simulink model "TCS"  (R2020a)
settings: Solver=VariableStepAuto  StartTime=0.0  StopTime=10.0  RelTol=1e-3
libraries: simulink x1
settings Model: Creator=Administrator  LastModifiedBy=Administrator

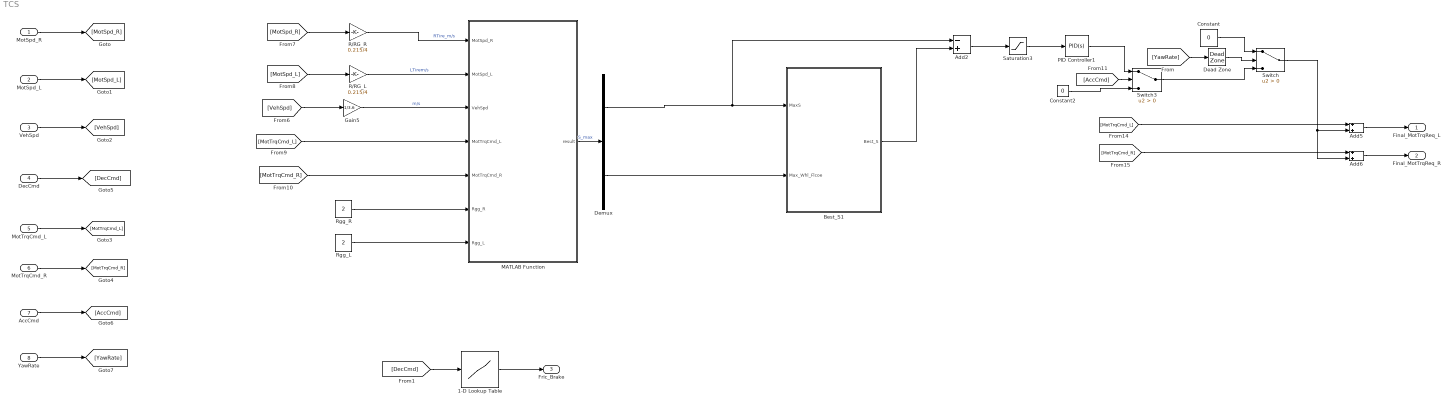
== system TCS ==
  MotSpd_R : Inport
  MotSpd_L : Inport  Port=2
  VehSpd : Inport  Port=3
  DecCmd : Inport  Port=4
  MotTrqCmd_L : Inport  Port=5
  MotTrqCmd_R : Inport  Port=6
  AccCmd : Inport  Port=7
  YawRate : Inport  Port=8
  1-D Lookup Table : Lookup_n-D  NumberOfTableDimensions=1  BreakpointsForDimension1=[0 , 0.2,0.4,0.6,0.8,1.0]  Table=[0 , 0.2,0.4,0.6,0.8,1.0]*60  InternalRulePriority=Speed  RndMeth=Simplest  InputSameDT=on
  Add2 : Sum  Inputs=-+
  Add5 : Sum
  Add6 : Sum
  Best_S1 : Subsystem
  Constant : Constant  Value=0
  Constant2 : Constant  Value=0
  Dead Zone : DeadZone  LowerValue=-0.25  UpperValue=0.25  SaturateOnIntegerOverflow=on
  Demux : Demux  Outputs=2
  Gain5 : Gain  Gain=1/3.6
  MATLAB Function : MATLAB Function  TreatAsAtomicUnit=on
  PID Controller1 : simulink/Continuous/PID Controller  Controller=PID  Form=Parallel  TimeDomain=Continuous-time  UseExternalTs=off  SampleTime=-1  IntegratorMethod=Forward Euler  FilterMethod=Forward Euler  ControllerParametersSource=internal  P=31  I=1  D=0  UseFilter=on  N=100  TunerSelectOption=Transfer Function Based (PID Tuner App)  InitialConditionSource=internal  InitialConditionForIntegrator=0  InitialConditionForFilter=0  DifferentiatorICPrevScaledInput=0  ExternalReset=none  TrackingMode=off  Kt=1  LimitOutput=off  UpperSaturationLimit=inf  LowerSaturationLimit=-inf  LinearizeAsGain=on  AntiWindupMode=none  Kb=1  POutMin=[]  POutMax=[]  IOutMin=[]  IOutMax=[]  DOutMin=[]  DOutMax=[]  NOutMin=[]  NOutMax=[]  SumOutMin=[]  SumOutMax=[]  SaturationOutMin=[]  SaturationOutMax=[]  PParamMin=[]  PParamMax=[]  IParamMin=[]  IParamMax=[]  DParamMin=[]  DParamMax=[]  NParamMin=[]  NParamMax=[]  KbParamMin=[]  KbParamMax=[]  KtParamMin=[]  KtParamMax=[]  KbOutMin=[]  KbOutMax=[]  KtOutMin=[]  KtOutMax=[]  IntegratorOutMin=[]  IntegratorOutMax=[]  FilterOutMin=[]  FilterOutMax=[]  SumI1OutMin=[]  SumI1OutMax=[]  SumI2OutMin=[]  SumI2OutMax=[]  SumI3OutMin=[]  SumI3OutMax=[]  SumI4OutMin=[]  SumI4OutMax=[]  SumDOutMin=[]  SumDOutMax=[]  DifferentiatorOutMin=[]  DifferentiatorOutMax=[]  FilterDiffOutCoefMin=[]  FilterDiffOutCoefMax=[]  ReciprocalOutMin=[]  ReciprocalOutMax=[]  SumDenOutMin=[]  SumDenOutMax=[]  SumNumOutMin=[]  SumNumOutMax=[]  DivideOutMin=[]  DivideOutMax=[]  UdiffTsProdOutMin=[]  UdiffTsProdOutMax=[]  NTsProdOutMin=[]  NTsProdOutMax=[]  UintegralTsProdOutMin=[]  UintegralTsProdOutMax=[]  UngainTsProdOutMin=[]  UngainTsProdOutMax=[]  IntegratorContinuousStateAttributes=''  IntegratorStateMustResolveToSignalObject=off  IntegratorRTWStateStorageClass=Auto  FilterContinuousStateAttributes=''  FilterStateMustResolveToSignalObject=off  FilterRTWStateStorageClass=Auto  ParallelPVariant=InternalParameters  IdealPVariant=Disabled  IVariant=InternalParameters  DVariant=InternalParameters  IntegratorVariant=Continuous  SatVariant=Disabled  AWVariant=Passthrough  PCopyVariant=Disabled  TRVariant=Disabled  FdbkBlocksVariant=Forward  IdealPFdbkVariant=Disabled  SatFdbkVariant=Disabled  DerivativeFilterVariant=ContFilter  NVariant=InternalParameters  NCopyVariant=Disabled  FilterICVariant=InternalICsFilter  IntegratorICVariant=InternalICs  ExternalResetVariant=Disabled  TRSumVariant=Passthrough  SumFdbkVariant=Disabled  SumVariant=Sum_PID  TsampFilterVariant=InternalTs  TsampNgainVariant=Passthrough  TsampIntegralVariant=Passthrough
  R/RG_L : Gain  Gain=0.215/4
  R/RG_R : Gain  Gain=0.215/4
  Rgg_L : Constant  Value=2
  Rgg_R : Constant  Value=2
  Saturation3 : Saturate  UpperLimit=2  LowerLimit=-2
  Switch : Switch  Criteria=u2 > Threshold
  Switch3 : Switch  Criteria=u2 > Threshold
  Final_MotTrqReq_L : Outport
  Final_MotTrqReq_R : Outport  Port=2
  Fric_Brake : Outport  Port=3
  wires:
  MotSpd_R/1 -> [MotSpd_R]
  MotSpd_L/1 -> [MotSpd_L]
  VehSpd/1 -> [VehSpd]
  MotTrqCmd_L/1 -> [MotTrqCmd_L]
  MotTrqCmd_R/1 -> [MotTrqCmd_R]
  DecCmd/1 -> [DecCmd]
  [VehSpd] -> Gain5/1
  [MotSpd_R] -> R/RG_R/1
  [MotSpd_L] -> R/RG_L/1
  R/RG_R/1 -> MATLAB Function/1(MotSpd_R)  "RTire_m/s"
  Gain5/1 -> MATLAB Function/3(VehSpd)  "m/s"
  R/RG_L/1 -> MATLAB Function/2(MotSpd_L)  "LTirem/s"
  Rgg_R/1 -> MATLAB Function/6(Rgg_R)
  Rgg_L/1 -> MATLAB Function/7(Rgg_L)
  [MotTrqCmd_L] -> MATLAB Function/4(MotTrqCmd_L)
  [MotTrqCmd_R] -> MATLAB Function/5(MotTrqCmd_R)
  Best_S1/1(Best_S) -> Add2/2
  Add2/1 -> Saturation3/1
  Saturation3/1 -> PID Controller1/1
  AccCmd/1 -> [AccCmd]
  [AccCmd] -> Switch3/2
  PID Controller1/1 -> Switch3/1
  Constant2/1 -> Switch3/3
  [MotTrqCmd_L] -> Add5/1
  [MotTrqCmd_R] -> Add6/1
  Add5/1 -> Final_MotTrqReq_L/1
  Add6/1 -> Final_MotTrqReq_R/1
  YawRate/1 -> [YawRate]
  Switch3/1 -> Switch/3
  Constant/1 -> Switch/1
  Switch/1 -> Add5/2, Add6/2
  [YawRate] -> Dead Zone/1
  Dead Zone/1 -> Switch/2
  1-D Lookup Table/1 -> Fric_Brake/1
  [DecCmd] -> 1-D Lookup Table/1
  MATLAB Function/1(result) -> Demux/1  "S_max"
  Demux/1 -> Add2/1, Best_S1/1(MaxS)
  Demux/2 -> Best_S1/2(Max_Whl_Flcoe)

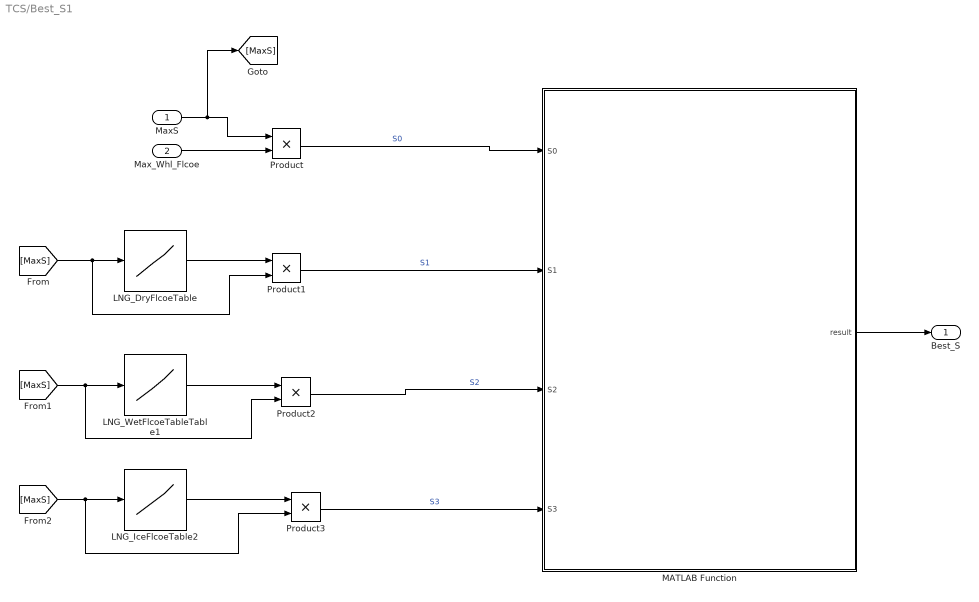
== system TCS/Best_S1 ==
  MaxS : Inport
  Max_Whl_Flcoe : Inport  Port=2
  LNG_DryFlcoeTable : Lookup_n-D  NumberOfTableDimensions=1  BreakpointsForDimension1="[0\t0.02\t0.04\t0.06\t0.08\t0.1\t0.12\t0.14\t0.16\t0.18\t0.2\t0.22\t0.24\t0.26\t0.28\t0.3\t0.32\t0.34\t0.36\t0.38\t0.4\t0.42\t0.44\t0.46\t0.48\t0.5\t0.52\t0.54\t0.56\t0.58\t0.6\t0.62\t0.64\t0.66\t0.68\t0.7\t0.72\t0.74\t0.76\t0.78\t0.8\t0.82\t0.84\t0.86\t0.88\t0.9\t0.92\t0.94\t0.96\t0.98\t1]"  Table="[0\t0.463\t0.738\t0.9\t0.994\t1.05\t1.07\t1.09\t1.09\t1.09\t1.08\t1.07\t1.06\t1.05\t1.04\t1.03\t1.02\t1.01\t1\t0.992\t0.981\t0.97\t0.959\t0.949\t0.938\t0.927\t0.916\t0.905\t0.895\t0.884\t0.873\t0.862\t0.851\t0.841\t0.83\t0.819\t0.808\t0.797\t0.787\t0.776\t0.765\t0.754\t0.743\t0.733\t0.722\t0.711\t0.7\t0.689\t0.679\t0.668\t0.657]"  InternalRulePriority=Speed  RndMeth=Simplest  InputSameDT=on
  LNG_IceFlcoeTable2 : Lookup_n-D  NumberOfTableDimensions=1  BreakpointsForDimension1=[ 0, 0.02, 0.04, 0.06, 0.08, 0.1, 0.12, 0.14, 0.16, 0.18, 0.2, 0.22, 0.24, 0.26, 0.28, 0.3, 0.32, 0.34, 0.36, 0.38, 0.4, 0.42, 0.44, 0.46, 0.48, 0.5, 0.52, 0.54, 0.56, 0.58, 0.6, 0.62, 0.64, 0.66, 0.68, 0.7, 0.72, 0.74, 0.76, 0.78, 0.8, 0.82, 0.84, 0.86, 0.88, 0.9, 0.92, 0.94, 0.96, 0.98, 1.0]  Table=[ 0, 0.05, 0.05, 0.05, 0.05, 0.05, 0.05, 0.05, 0.05, 0.05, 0.05, 0.05, 0.05, 0.05, 0.05, 0.05, 0.05, 0.05, 0.05, 0.05, 0.05, 0.05, 0.05, 0.05, 0.05, 0.05, 0.05, 0.05, 0.049, 0.049, 0.049, 0.049, 0.049, 0.049, 0.049, 0.049, 0.049, 0.049, 0.049, 0.049, 0.049, 0.049, 0.049, 0.049, 0.049, 0.049, 0.049, 0.049, 0.049, 0.049, 0.049]  InternalRulePriority=Speed  RndMeth=Simplest  InputSameDT=on
  LNG_WetFlcoeTableTable1 : Lookup_n-D  NumberOfTableDimensions=1  BreakpointsForDimension1=[ 0, 0.02, 0.04, 0.06, 0.08, 0.1, 0.12, 0.14, 0.16, 0.18, 0.2, 0.22, 0.24, 0.26, 0.28, 0.3, 0.32, 0.34, 0.36, 0.38, 0.4, 0.42, 0.44, 0.46, 0.48, 0.5, 0.52, 0.54, 0.56, 0.58, 0.6, 0.62, 0.64, 0.66, 0.68, 0.7, 0.72, 0.74, 0.76, 0.78, 0.8, 0.82, 0.84, 0.86, 0.88, 0.9, 0.92, 0.94, 0.96, 0.98, 1.0]  Table=[ 0, 0.41, 0.62, 0.72, 0.77, 0.79, 0.8, 0.8, 0.8, 0.79, 0.79, 0.78, 0.77, 0.77, 0.76, 0.75, 0.74, 0.74, 0.73, 0.72, 0.72, 0.71, 0.7, 0.7, 0.69, 0.68, 0.68, 0.67, 0.66, 0.65, 0.65, 0.64, 0.63, 0.63, 0.62, 0.61, 0.6, 0.6, 0.59, 0.58, 0.58, 0.57, 0.56, 0.56, 0.55, 0.54, 0.54, 0.53, 0.52, 0.51, 0.51]  InternalRulePriority=Speed  RndMeth=Simplest  InputSameDT=on
  MATLAB Function : MATLAB Function  TreatAsAtomicUnit=on
  Product{,1..3} (4 alike) : Product
  Best_S : Outport
  wires:
  Product3/1 -> MATLAB Function/4(S3)  "S3"
  Product2/1 -> MATLAB Function/3(S2)  "S2"
  Product1/1 -> MATLAB Function/2(S1)  "S1"
  Product/1 -> MATLAB Function/1(S0)  "S0"
  LNG_IceFlcoeTable2/1 -> Product3/1
  LNG_WetFlcoeTableTable1/1 -> Product2/1
  LNG_DryFlcoeTable/1 -> Product1/1
  [MaxS] -> LNG_WetFlcoeTableTable1/1, Product2/2
  [MaxS] -> LNG_IceFlcoeTable2/1, Product3/2
  [MaxS] -> LNG_DryFlcoeTable/1, Product1/2
  Max_Whl_Flcoe/1 -> Product/2
  MaxS/1 -> Product/1, [MaxS]
  MATLAB Function/1(result) -> Best_S/1

== matlab function TCS/MATLAB Function ==
  data: MotSpd_R input; result output double size=2; MotSpd_L input; VehSpd input; MotTrqCmd_L input; MotTrqCmd_R input; Rgg_R input; Rgg_L input
function result = fcn(MotSpd_R,MotSpd_L,VehSpd,MotTrqCmd_L,MotTrqCmd_R,Rgg_R,Rgg_L)
S_r = (MotSpd_R - VehSpd)/MotSpd_R;
S_l = (MotSpd_L - VehSpd)/MotSpd_L;
 if(S_r>S_l)
     S_max = S_r;
     u_max = (MotTrqCmd_R*Rgg_R*0.95)/0.215/(330*0.55*0.5);
 else
     S_max = S_l;
     u_max = (MotTrqCmd_L*Rgg_L*0.95)/0.215/(330*0.55*0.5);
 end
result = [S_max;u_max];
end

== matlab function TCS/Best_S1/MATLAB Function ==
  data: S0 input; result output; S1 input; S2 input; S3 input
function result = fcn(S0,S1,S2,S3)
    a = abs(S0-S1);a1=0.16;
    b=abs(S0-S2);b1=0.131;
    c = abs(S0-S3);c1=0.031;
    if a>b
        if b>c
            best_S = c1;
        else
            best_S =b1;
        end
    else
       if a>c
           best_S = c1;
       else
           best_S = a1;
       end
    end
result = best_S;
end
